simulink model "Ref42_SFPPC_compare"  (R2025b)
settings: Solver=ode4  StartTime=0.0  StopTime=20  FixedStep=0.001  RelTol=1e-3
settings Model: Creator=31586  LastModifiedBy=31586

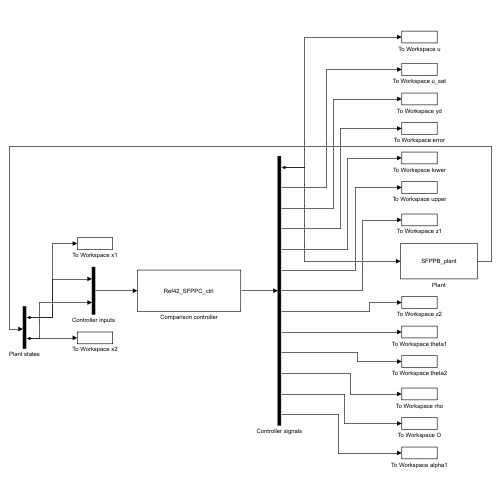
[thumbnail: Simulink's stored preview of the top-level diagram]
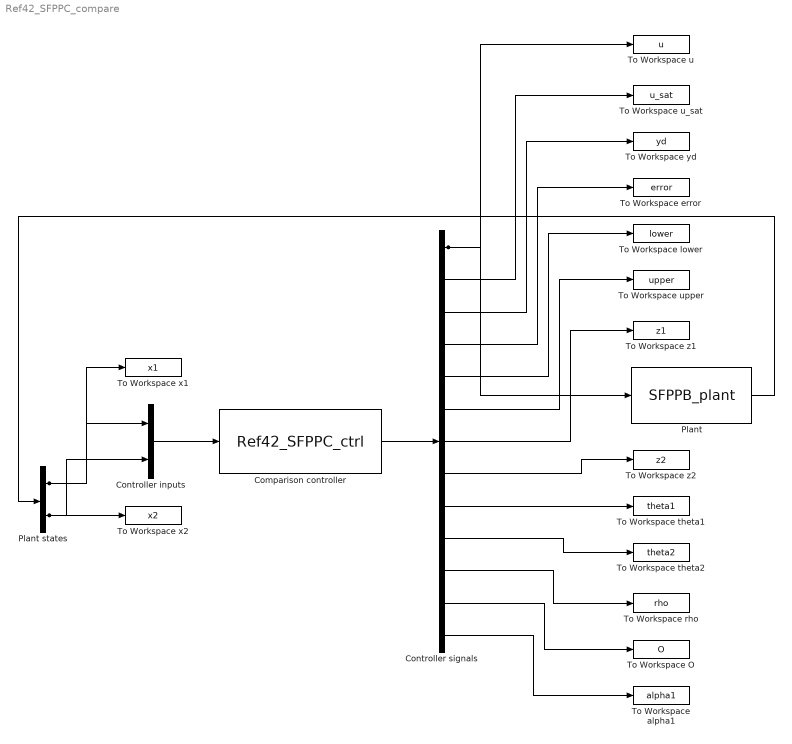
== system Ref42_SFPPC_compare ==
  Comparison controller : S-Function  FunctionName=Ref42_SFPPC_ctrl  SFunctionDeploymentMode=off  EnableBusSupport=off
  Controller inputs : Mux  Inputs=2
  Controller signals : Demux  Outputs=13
  Plant : S-Function  FunctionName=SFPPB_plant  SFunctionDeploymentMode=off  EnableBusSupport=off
  Plant states : Demux  Outputs=2
  To Workspace O : ToWorkspace  VariableName=O  SaveFormat=Timeseries  SampleTime=-1
  To Workspace alpha1 : ToWorkspace  VariableName=alpha1  SaveFormat=Timeseries  SampleTime=-1
  To Workspace error : ToWorkspace  VariableName=error  SaveFormat=Timeseries  SampleTime=-1
  To Workspace lower : ToWorkspace  VariableName=lower  SaveFormat=Timeseries  SampleTime=-1
  To Workspace rho : ToWorkspace  VariableName=rho  SaveFormat=Timeseries  SampleTime=-1
  To Workspace theta1 : ToWorkspace  VariableName=theta1  SaveFormat=Timeseries  SampleTime=-1
  To Workspace theta2 : ToWorkspace  VariableName=theta2  SaveFormat=Timeseries  SampleTime=-1
  To Workspace u : ToWorkspace  VariableName=u  SaveFormat=Timeseries  SampleTime=-1
  To Workspace u_sat : ToWorkspace  VariableName=u_sat  SaveFormat=Timeseries  SampleTime=-1
  To Workspace upper : ToWorkspace  VariableName=upper  SaveFormat=Timeseries  SampleTime=-1
  To Workspace x1 : ToWorkspace  VariableName=x1  SaveFormat=Timeseries  SampleTime=-1
  To Workspace x2 : ToWorkspace  VariableName=x2  SaveFormat=Timeseries  SampleTime=-1
  To Workspace yd : ToWorkspace  VariableName=yd  SaveFormat=Timeseries  SampleTime=-1
  To Workspace z1 : ToWorkspace  VariableName=z1  SaveFormat=Timeseries  SampleTime=-1
  To Workspace z2 : ToWorkspace  VariableName=z2  SaveFormat=Timeseries  SampleTime=-1
  wires:
  Plant states/2 -> To Workspace x2/1, Controller inputs/2
  Plant states/1 -> Controller inputs/1, To Workspace x1/1
  Controller inputs/1 -> Comparison controller/1
  Controller signals/10 -> To Workspace theta2/1
  Controller signals/8 -> To Workspace z2/1
  Controller signals/6 -> To Workspace upper/1
  Controller signals/4 -> To Workspace error/1
  Comparison controller/1 -> Controller signals/1
  Controller signals/1 -> Plant/1, To Workspace u/1
  Controller signals/3 -> To Workspace yd/1
  Controller signals/2 -> To Workspace u_sat/1
  Controller signals/11 -> To Workspace rho/1
  Controller signals/9 -> To Workspace theta1/1
  Controller signals/7 -> To Workspace z1/1
  Controller signals/5 -> To Workspace lower/1
  Controller signals/12 -> To Workspace O/1
  Controller signals/13 -> To Workspace alpha1/1
  Plant/1 -> Plant states/1
